simulink model "series_shunt_2a"  (Simulink 7.4)
settings: Solver=ode23tb  StartTime=0.0  StopTime=100e-6  MaxStep=10e-9  RelTol=1e-4
InitFcn:
  | series_shunt_2c;
StopFcn:
  | if ~SPECTRUM_FLAG
  |      %% plot measured sparameters using RFTB
  |     amp=rfdata.data;
  |     amp.Freq=spar(:,1);
  | %%
  |     amp.S_parameters=complex(zeros(2,2,length(amp.Freq)));
  |    if spar(1,6)==1
  |       amp.S_Parameters(1,1,:)=spar(:,2)+1i*spar(:,3);
  |       amp.S_Parameters(2,1,:)=spar(:,4)+1i*spar(:,5);
  |       subplot(2,1,1);
  |       hplot1= smith(amp,'s11')
  |       subplot(2,1,2);
  |       hplot2 = plot(amp,'s21');
  |       axis([amp.Freq(1)/1e6,amp.Freq(end)/1e6,0,20]);
  |    else
  |       amp.S_Parameters(2,2,:)=spar(:,2)+1i*spar(:,3);
  |       amp.S_Parameters(1,2,:)=spar(:,4)+1i*spar(:,5);
  |       subplot(2,1,1);
  |       hplot1= smith(amp,'s22')
  |       subplot(2,1,2);
  |       hplot2 = plot(amp,'s12');
  |    end;
  | end
values from neighbouring files (symbols this model uses):
  Base_Bias = 0.8    [series_shunt_2c.m]
  Beta = 100    [series_shunt_2c.m]
  Cbc = 10e-12    (= 1e-11)    [series_shunt_2c.m]
  Cbe = 250e-12    (= 2.5e-10)    [series_shunt_2c.m]
  ICs = IEs    (= 1e-12)    [series_shunt_2c.m]
  IEs = 1e-12    [series_shunt_2c.m]
  Lpri_1 = 5e-6    (= 5e-06)    [series_shunt_2c.m]
  Lsec_1 = Lpri_1*Tr_1^2    [series_shunt_2c.m]
  M12_1 = K*Tr_1*Lpri_1    [series_shunt_2c.m]
  M13_1 = M12_1    [series_shunt_2c.m]
  M23_1 = K*Lsec_1    [series_shunt_2c.m]
  Rbb = 5    [series_shunt_2c.m]
  Re = (Rl^2)/Rfb    (= 1.52007654004)    [series_shunt_2c.m]
  Rfb = Rl*(1*Av+1)    (= 81.21748272)    [series_shunt_2c.m]
  Rloss = .1    (= 0.1)    [series_shunt_2c.m]
  Vcc = 12    [series_shunt_2c.m]
undefined symbols (not defined in the file or in its folder): Fs, magnitude, One, sided
libraries: powerlib x52, dspindex x12, dspsigops x6, dsparch4 x5, simulink x4, dspbuff3 x4, dspxfrm3 x4, dsparch3 x4, dspsnks4 x3, dspmtrx3 x2
(part 2 of 2)

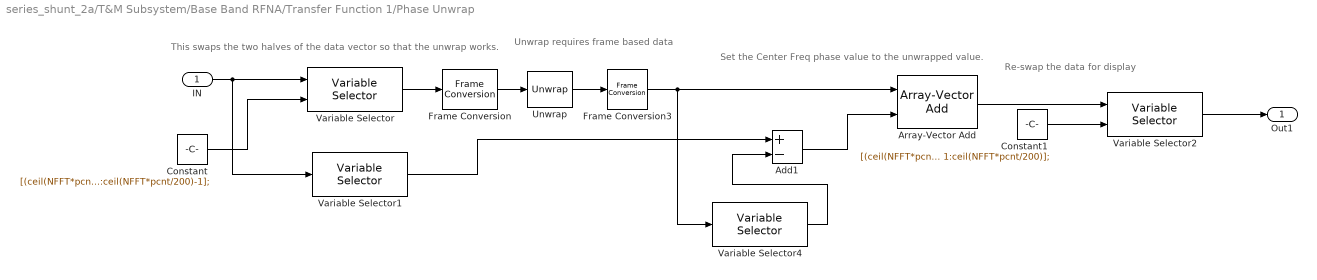
== system series_shunt_2a/T&M Subsystem/Base Band RFNA/Transfer Function 1/Phase Unwrap ==
  note: This swaps the two halves of the data vector
      | so that the unwrap works.
  note: Set the Center Freq phase value to the unwrapped value.
  note: Re-swap the data for display
  note: Unwrap requires frame based data
  IN : Inport  OutDataType=sfix(16)  OutScaling=2^0
  Add1 : Sum  Inputs=+-  OutDataType=sfix(16)  OutScaling=2^-10
  Array-Vector Add : dspmtrx3/Array-Vector Add  DialogController=dspDDGCreate  DialogControllerArgs=DataTag9  Dimension=2  V_Source=Input port  V_VectFromMask=[0.5 0.25]  firstCoeffDataTypeStr=Inherit: Same word length as input  firstCoeffLastDataTypeStr=Inherit: Same word length as input  firstCoeffMin=[]  firstCoeffMax=[]  outputDataTypeStr=Inherit: Same as accumulator  outputLastDataTypeStr=Inherit: Same as accumulator  outputMin=[]  outputMax=[]  roundingMode=Floor  overflowMode=off
  Constant : Constant  Value=[(ceil(NFFT*pcnt/200)):ceil(NFFT*pcnt/100) 1:ceil(NFFT*pcnt/200)-1];  OutDataType=sfix(16)  OutScaling=2^0
  Constant1 : Constant  Value=[(ceil(NFFT*pcnt/200)+1):ceil(NFFT*pcnt/100) 1:ceil(NFFT*pcnt/200)];  OutDataType=sfix(16)  OutScaling=2^0
  Frame Conversion : FrameConversion
  Frame Conversion3 : FrameConversion  OutFrame=Sample-based
  Unwrap : dspsigops/Unwrap  running=on  tol=pi
  Variable Selector : dspindex/Variable Selector  NumInputs=1  rowsOrCols=Rows  IdxMode=Variable  Elements=[1 3]  ZerOneIdxMode=One-based  errmode=Clip Index  FillMode=on  FillValues=0
  Variable Selector1 : dspindex/Variable Selector  NumInputs=1  rowsOrCols=Rows  IdxMode=Fixed  Elements=[1]  ZerOneIdxMode=One-based  errmode=Clip Index  FillMode=on  FillValues=0
  Variable Selector2 : dspindex/Variable Selector  NumInputs=1  rowsOrCols=Rows  IdxMode=Variable  Elements=[1 3]  ZerOneIdxMode=One-based  errmode=Clip Index  FillMode=on  FillValues=0
  Variable Selector4 : dspindex/Variable Selector  NumInputs=1  rowsOrCols=Rows  IdxMode=Fixed  Elements=length([(ceil(NFFT*pcnt/200)+1):ceil(NFFT*pcnt/100) 1:ceil(NFFT*pcnt/200)] )/2+1  ZerOneIdxMode=One-based  errmode=Clip Index  FillMode=on  FillValues=0
  Out1 : Outport  OutDataType=sfix(16)  OutScaling=2^0
  wires:
  Frame Conversion/1 -> Unwrap/1
  Variable Selector2/1 -> Out1/1
  IN/1 -> Variable Selector/1, Variable Selector1/1
  Constant/1 -> Variable Selector/2
  Variable Selector/1 -> Frame Conversion/1
  Variable Selector1/1 -> Add1/1
  Unwrap/1 -> Frame Conversion3/1
  Variable Selector4/1 -> Add1/2
  Constant1/1 -> Variable Selector2/2
  Frame Conversion3/1 -> Variable Selector4/1, Array-Vector Add/1
  Add1/1 -> Array-Vector Add/2
  Array-Vector Add/1 -> Variable Selector2/1
